simulink model "pmsm_paper_sfunction"  (R2021b)
settings: Solver=ode23t  StartTime=0.0  StopTime=0.4  RelTol=1e-3  EnableMultiTasking=on
InitFcn:
  | Ts=50e-6;
  | Ld = 8.5e-3;
  | R = 2.875;
undefined symbols (not defined in the file or in its folder): lambda, Lq, Pn
libraries: powerlib_extras x3, spsdq0toabcLib x1, spspowerguiLib x1
settings Model: Creator=Administrator  LastModifiedBy=wkw
settings SolverCC: AlgebraicLoopSolver=TrustRegion
settings DataIOCC: LimitDataPoints=on  SaveFormat=Array  SignalLoggingSaveFormat=ModelDataLogs  ReturnWorkspaceOutputs=off
settings OptimizationCC: ExpressionDepthLimit=2147483647  InitFltsAndDblsToZero=on  LifeSpan=inf
settings DebuggingCC: SaveWithParameterizedLinksMsg=none  UnderspecifiedInitializationDetection=Classic  MergeDetectMultiDrivingBlocksExec=none  SolverPrmCheckMsg=warning  FcnCallInpInsideContextMsg=warning  StateNameClashWarn=warning  SFUnexpectedBacktrackingDiag=warning  SFNoUnconditionalDefaultTransitionDiag=warning  SFExecutionAtInitializationDiag=none  SFMachineParentedDataDiag=warning  ArithmeticOperatorsInVariantConditions=warning
settings HardwareCC: ProdBitPerPointer=32  ProdBitPerSizeT=32  ProdBitPerPtrDiffT=32  ProdLargestAtomicFloat=None  ProdIntDivRoundTo=Undefined  ProdEndianess=Unspecified  ProdWordSize=32  ProdHWDeviceType=32-bit Generic
settings ModelReferenceCC: PropagateSignalLabelsOutOfModel=off
settings SFSimCC: SimUseLocalCustomCode=off  CustomCodeUndefinedFunction=UseInterfaceOnly
settings RTWCC: RTWUseLocalCustomCode=off
settings CodeAppCC: StateflowObjectComments=on
settings GRTTargetCC: TargetFcnLib=ansi_tfl_tmw.mat  TargetLangStandard=C89/C90 (ANSI)  CombineOutputUpdateFcns=off  GRTInterface=on
settings ConfigComp: CovMetricSettings=dw  CovSaveCumulativeToWorkspaceVar=on  CovSaveSingleToWorkspaceVar=on  CovExternalEMLEnable=off

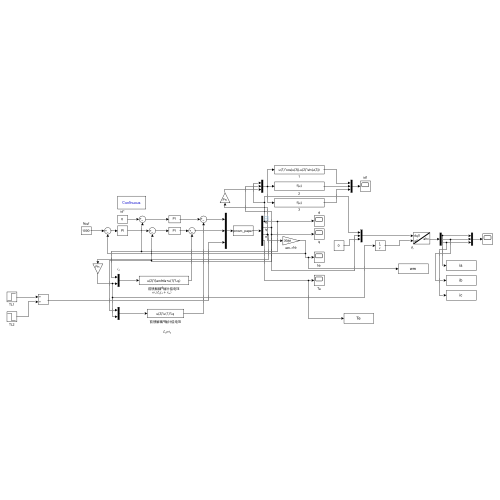
[thumbnail: Simulink's stored preview of the top-level diagram]
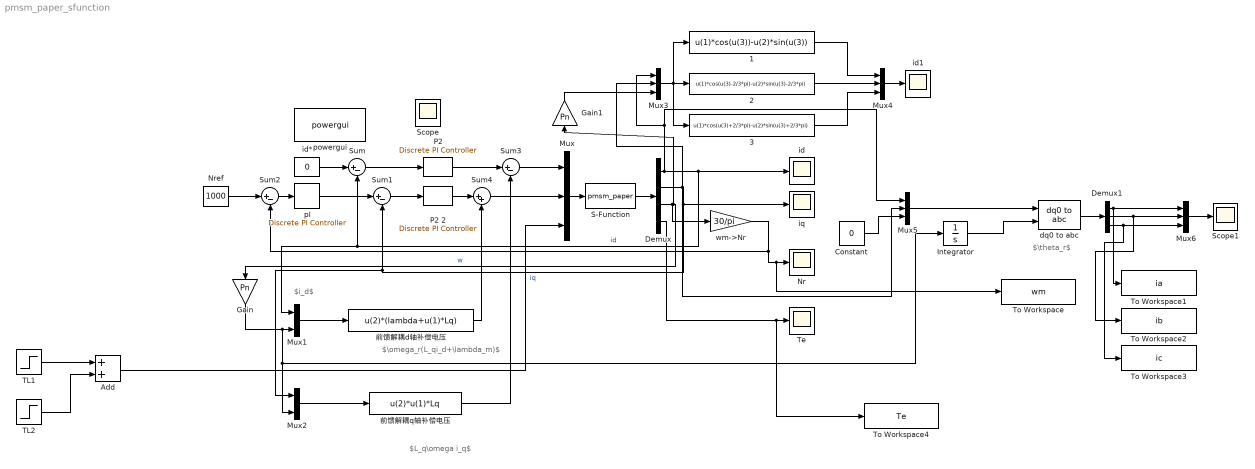
== system pmsm_paper_sfunction ==
  note: $\theta_r$
  note: $i_d$
  note: $\omega_r(L_qi_d+\lambda_m)$
  note: $L_q\omega i_q$
  1 : Fcn  Expr=u(1)*cos(u(3))-u(2)*sin(u(3))
  2 : Fcn  Expr=u(1)*cos(u(3)-2/3*pi)-u(2)*sin(u(3)-2/3*pi)
  3 : Fcn  Expr=u(1)*cos(u(3)+2/3*pi)-u(2)*sin(u(3)+2/3*pi)
  Add : Sum
  Constant : Constant  Value=0
  Demux : Demux
  Demux1 : Demux  Outputs=3
  Gain : Gain  Gain=Pn
  Gain1 : Gain  Gain=Pn
  Integrator : Integrator
  Mux{,3..6} (5 alike) : Mux  Inputs=3
  Mux1 : Mux  Inputs=2
  Mux2 : Mux  Inputs=2
  Nr : Scope
  Nref : Constant  Value=1000
  "P2 " : powerlib_extras/Discrete  Control Blocks/Discrete PI Controller  Kp=0.2  Ki=0.06  Par_Limits=[250 -250]  Init=0  Ts=Ts
  P2 2 : powerlib_extras/Discrete  Control Blocks/Discrete PI Controller  Kp=0.2  Ki=0.06  Par_Limits=[250 -250]  Init=0  Ts=Ts
  S-Function : S-Function  FunctionName=pmsm_paper  SFunctionDeploymentMode=off  EnableBusSupport=off
  Scope1 : Scope
  Sum{,1..3} (4 alike) : Sum  Inputs=|+-
  Sum4 : Sum  Inputs=|++
  TL1 : Step  Time=0.2  After=1.27  SampleTime=0
  TL2 : Step  Time=0.3  After=-0.62  SampleTime=0
  Te : Scope
  To Workspace : ToWorkspace  VariableName=wm  SaveFormat=Timeseries  SampleTime=-1
  To Workspace1 : ToWorkspace  VariableName=ia  SaveFormat=Timeseries  SampleTime=-1
  To Workspace2 : ToWorkspace  VariableName=ib  SaveFormat=Timeseries  SampleTime=-1
  To Workspace3 : ToWorkspace  VariableName=ic  SaveFormat=Timeseries  SampleTime=-1
  To Workspace4 : ToWorkspace  VariableName=Te  SaveFormat=Timeseries  SampleTime=-1
  dq0 to abc : spsdq0toabcLib/dq0 to abc  Alignment=90 degrees behind phase A axis
  id : Scope
  id* : Constant  Value=0
  id1 : Scope
  iq : Scope
  "pI " : powerlib_extras/Discrete  Control Blocks/Discrete PI Controller  Kp=0.11  Ki=15  Par_Limits=[300 -300]  Init=0  Ts=Ts
  powergui : spspowerguiLib/powergui  SimulationMode=Continuous  SampleTime=50e-6  frequency=60  Iterations=50  frequencyindice=0  Pbase=100e6  ErrMax=1e-4  UnitsV=kV  UnitsW=MW  buscounter=0  FunctionMessages=off  echomessages=off  EnableUseOfTLC=off  CurrentSourceSwitches=on  DisableSnubberDevices=off  DisableRonSwitches=off  DisableVfSwitches=off  DisplayEquations=off  AutomaticDiscreteSolvers=off  SolverType=Tustin/Backward Euler (TBE)  Interpol=off  ExternalGateDelay=off  methode=off  Ts=0  x0status=blocks  SPID=off  SwTol=0  HookPort=off  NonlinearTolerance=1e-4  nMaxIteration=100  ContinueOnMaxIteration=off  RestoreLinks=warning  ResistiveCurrentMeasurement=off  Frange=[0:2:500]  Ylog=off  Xlog=on  ShowGrid=off  save=off  variable=ZData  structure=0  ZoomFFT=off  StartTime=0.0  cycles=1  DisplayStyle=1  fundamental=60  FreqAxis=off  MaxFrequency=1000  frequencyindicesteady=1  RmsSteady=1  display=off
  wm->Nr : Gain  Gain=30/pi
  前馈解耦d轴补偿电压 : Fcn  Expr=u(2)*(lambda+u(1)*Lq)
  前馈解耦q轴补偿电压 : Fcn  Expr=u(2)*u(1)*Lq
  Scope : Scope
  wires:
  Sum1/1 -> P2 2/1
  "pI "/1 -> Sum1/1
  Sum2/1 -> "pI "/1
  wm->Nr/1 -> To Workspace/1, Nr/1, Sum2/2
  Nref/1 -> Sum2/1
  Demux/1 -> Mux5/1, Mux3/1, id/1, Mux1/1, Sum/2  "id"
  Demux/2 -> Mux3/2, iq/1, Mux2/1, Sum1/2, Mux5/2  "iq"
  P2 2/1 -> Sum4/1
  "P2 "/1 -> Sum3/1
  Demux/3 -> Gain1/1, Gain/1, wm->Nr/1  "w"
  Add/1 -> Mux/3
  Mux/1 -> S-Function/1
  S-Function/1 -> Demux/1
  Sum/1 -> "P2 "/1
  id*/1 -> Sum/1
  Demux/4 -> To Workspace4/1, Te/1
  TL1/1 -> Add/1
  TL2/1 -> Add/2
  Mux1/1 -> 前馈解耦d轴补偿电压/1
  Gain/1 -> Integrator/1, Mux2/2, Mux1/2
  Sum3/1 -> Mux/1
  Sum4/1 -> Mux/2
  前馈解耦d轴补偿电压/1 -> Sum4/2
  Mux2/1 -> 前馈解耦q轴补偿电压/1
  前馈解耦q轴补偿电压/1 -> Sum3/2
  Mux3/1 -> 3/1, 1/1, 2/1
  Gain1/1 -> Mux3/3
  Mux4/1 -> id1/1
  1/1 -> Mux4/1
  2/1 -> Mux4/2
  3/1 -> Mux4/3
  Mux5/1 -> dq0 to abc/1
  Constant/1 -> Mux5/3
  dq0 to abc/1 -> Demux1/1
  Integrator/1 -> dq0 to abc/2
  Demux1/2 -> To Workspace2/1, Mux6/2
  Mux6/1 -> Scope1/1
  Demux1/1 -> To Workspace1/1, Mux6/1
  Demux1/3 -> To Workspace3/1, Mux6/3
